simulink model "RBDmodel"  (R2023a)
settings: Solver=ode15s  StartTime=0.0  StopTime=4  FixedStep=0.0001  RelTol=1e-3  AbsTol=1e-3  EnableMultiTasking=on
model workspace (MAT data in the model file):
  C_Gimbal = 0.5
  C_IAP = 0.01
  IAP_Pa = 0
  K_Gimbal = 0
  K_IAP = 200
  LeftAbdominalMuscleForce = 0
  LeftBackMuscleForce = 0
  LeftTransverse1MuscleForce = 0
  LeftTransverse2MuscleForce = 0
  Moment_AR = 0
  Moment_FE = 7.5
  Moment_LB = 0
  RightAbdominalMuscleForce = 0
  RightBackMuscleForce = 0
  RightTransverse1MuscleForce = 0
  RightTransverse2MuscleForce = 0
  a = 1
  b = 1
  muscle_color = [0 0 1]
  muscle_radius = 1
undefined symbols (not defined in the file): X, Y, Z
libraries: nesl_utility x346, sm_lib x329, simulink_extras x33, checkpacklib x3, simulink x1
(part 1 of 12)
settings Model: PacingRate=0.110000  Creator=Siril TD  LastModifiedBy=siril
settings SolverCC: ZeroCrossAlgorithm=Adaptive  AutoInsertRateTranBlk=on
settings DataIOCC: LimitDataPoints=on  MaxDataPoints=50000  ReturnWorkspaceOutputsName=SDOSimTest_Log
settings OptimizationCC: LifeSpan=inf
settings DebuggingCC: IgnoredZcDiagnostic=none  UnconnectedInputMsg=warning  UnconnectedOutputMsg=warning  UnconnectedLineMsg=warning  AllowSymbolicDim=off  SFUnexpectedBacktrackingDiag=warning  SFNoUnconditionalDefaultTransitionDiag=warning  SFExecutionAtInitializationDiag=none  ArithmeticOperatorsInVariantConditions=warning
settings ModelReferenceCC: EnableRefExpFcnMdlSchedulingChecks=on
settings SFSimCC: SimUseLocalCustomCode=off  CustomCodeUndefinedFunction=UseInterfaceOnly
settings RTWCC: RTWUseLocalCustomCode=off  DLArmComputeVersion=19.05
settings CodeAppCC: StateflowObjectComments=on
settings GRTTargetCC: TargetLangStandard=C89/C90 (ANSI)
settings ConfigComp: CovMetricSettings=dw  CovSaveCumulativeToWorkspaceVar=on  CovSaveSingleToWorkspaceVar=on  CovExternalEMLEnable=off  CovSFcnEnable=off
settings SimscapeCC: SimscapeLogType=all  SimscapeLogSimulationStatistics=on  SimscapeLogDataHistory=10000

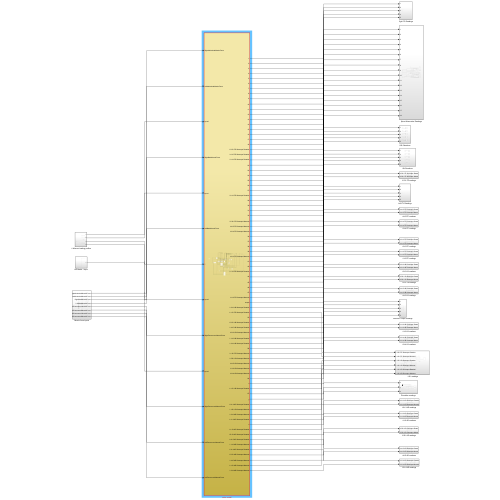
[thumbnail: Simulink's stored preview of the top-level diagram]
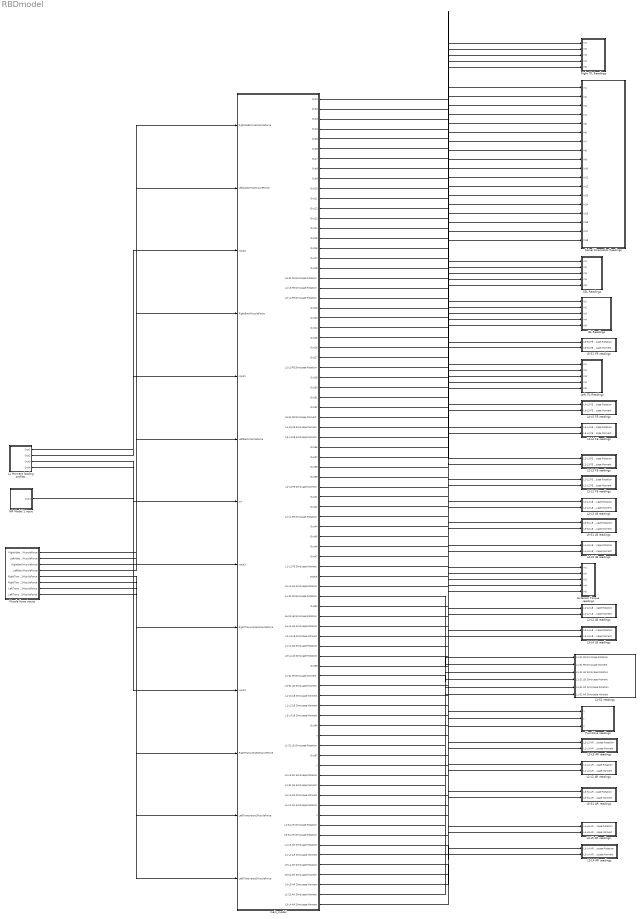
== system RBDmodel ==
  Extensor Torque readings : Subsystem
  IAP Model 1 input : Subsystem
  ISL Readings : Subsystem
  L1 Moment loading profiles : Subsystem
  L1-L2 AR readings : Subsystem
  L1-L2 FE readings : Subsystem
  L1-L2 LB readings : Subsystem
  L1-S1 readings : Subsystem
  L2-L3 AR readings : Subsystem
  L2-L3 FE readings : Subsystem
  L2-L3 LB readings : Subsystem
  L3-L4 AR readings : Subsystem
  L3-L4 FE readings : Subsystem
  L3-L4 LB readings : Subsystem
  L4-L5 AR readings : Subsystem
  L4-L5 FE readings : Subsystem
  L4-L5 LB readings : Subsystem
  L5-S1 AR readings : Subsystem
  L5-S1 FE readings : Subsystem
  L5-S1 LB readings : Subsystem
  Left ITL Readings : Subsystem
  Muscle force inputs : Subsystem
  Plumbline readings : Subsystem
  Right ITL Readings : Subsystem
  SSL Readings : Subsystem
  Spinal Kinematics Readings : Subsystem
  main_model : Subsystem  TreatAsAtomicUnit=on
  wires:
  main_model/20(L4-L5 FE Simscape Rotation) -> L4-L5 FE readings/1(L4-L5 FE Simscape Rotation)
  main_model/67(Out67) -> Extensor Torque readings/5(In5)
  Muscle force inputs/4(LeftBackMuscleForce) -> main_model/6(LeftBackMuscleForce)
  Muscle force inputs/3(RightBackMuscleForce) -> main_model/4(RightBackMuscleForce)
  L1 Moment loading profiles/1(Out1) -> main_model/3(input0)
  main_model/31(Out31) -> SSL Readings/4(In4)
  main_model/81(L1-S1 AR Simscape Moment) -> L1-S1 readings/6(L1-S1 AR Simscape Moment)
  main_model/56(L1-L2 LB Simscape Rotation) -> L1-L2 LB readings/1(L1-L2 LB Simscape Rotation)
  L1 Moment loading profiles/2(Out2) -> main_model/5(input1)
  L1 Moment loading profiles/3(Out3) -> main_model/8(input2)
  main_model/50(L2-L3 LB Simscape Rotation) -> L2-L3 LB readings/1(L2-L3 LB Simscape Rotation)
  main_model/6(Out6) -> SSL Readings/1(In1)
  L1 Moment loading profiles/4(Out4) -> main_model/10(input3)
  Muscle force inputs/1(RightAbdominalMuscleForce) -> main_model/1(RightAbdominalMuscleForce)
  main_model/16(Out16) -> Left ITL Readings/2(In2)
  IAP Model 1 input/1(Out1) -> main_model/7(In7)
  Muscle force inputs/2(LeftAbdominalMuscleForce) -> main_model/2(LeftAbdominalMuscleForce)
  Muscle force inputs/5(RightTransverse1MuscleForce) -> main_model/9(RightTransverse1MuscleForce)
  Muscle force inputs/6(RightTransverse2MuscleForce) -> main_model/11(RightTransverse2MuscleForce)
  main_model/62(L1-L2 LB Simscape Moment) -> L1-L2 LB readings/2(L1-L2 LB Simscape Moment)
  Muscle force inputs/8(LeftTransverse2MuscleForce) -> main_model/13(LeftTransverse2MuscleForce)
  Muscle force inputs/7(LeftTransverse1MuscleForce) -> main_model/12(LeftTransverse1MuscleForce)
  main_model/63(L3-L4 LB Simscape Moment) -> L3-L4 LB readings/2(L3-L4 LB Simscape Moment)
  main_model/1(Out1) -> Spinal Kinematics Readings/1(In1)
  main_model/30(Out30) -> Spinal Kinematics Readings/13(In13)
  main_model/2(Out2) -> Spinal Kinematics Readings/2(In2)
  main_model/13(Out13) -> SSL Readings/2(In2)
  main_model/21(L3-L4 FE Simscape Rotation) -> L3-L4 FE readings/1(L3-L4 FE Simscape Rotation)
  main_model/3(Out3) -> ISL Readings/1(In1)
  main_model/44(Out44) -> Spinal Kinematics Readings/17(In17)
  main_model/25(Out25) -> Spinal Kinematics Readings/11(In11)
  main_model/79(L5-S1 AR Simscape Moment) -> L5-S1 AR readings/2(L5-S1 AR Simscape Moment)
  main_model/4(Out4) -> Spinal Kinematics Readings/3(In3)
  main_model/5(Out5) -> Spinal Kinematics Readings/4(In4)
  main_model/77(L1-L2 AR Simscape Moment) -> L1-L2 AR readings/2(L1-L2 AR Simscape Moment)
  main_model/36(Out36) -> Spinal Kinematics Readings/14(In14)
  main_model/78(L3-L4 AR Simscape Rotation) -> L3-L4 AR readings/1(L3-L4 AR Simscape Rotation)
  main_model/26(Out26) -> Left ITL Readings/3(In3)
  main_model/7(Out7) -> Spinal Kinematics Readings/5(In5)
  main_model/18(Out18) -> Right ITL Readings/3(In3)
  main_model/8(Out8) -> Left ITL Readings/1(In1)
  main_model/9(Out9) -> Right ITL Readings/1(In1)
  main_model/10(Out10) -> Spinal Kinematics Readings/6(In6)
  main_model/11(Out11) -> ISL Readings/2(In2)
  main_model/12(Out12) -> Spinal Kinematics Readings/7(In7)
  main_model/38(Out38) -> Left ITL Readings/4(In4)
  main_model/14(Out14) -> Right ITL Readings/2(In2)
  main_model/15(Out15) -> Spinal Kinematics Readings/8(In8)
  main_model/17(Out17) -> Spinal Kinematics Readings/9(In9)
  main_model/27(Out27) -> Right ITL Readings/4(In4)
  main_model/19(L5-S1 FE Simscape Rotation) -> L5-S1 FE readings/1(L5-S1 FE Simscape Rotation)
  main_model/22(Out22) -> Spinal Kinematics Readings/10(In10)
  main_model/33(L5-S1 FE Simscape Moment) -> L5-S1 FE readings/2(L5-S1 FE Simscape Moment)
  main_model/23(Out23) -> ISL Readings/3(In3)
  main_model/45(Out45) -> Left ITL Readings/5(In5)
  main_model/24(Out24) -> SSL Readings/3(In3)
  main_model/28(L2-L3 FE Simscape Rotation) -> L2-L3 FE readings/1(L2-L3 FE Simscape Rotation)
  main_model/29(Out29) -> Spinal Kinematics Readings/12(In12)
  main_model/32(Out32) -> Right ITL Readings/5(In5)
  main_model/34(L4-L5 FE Simscape Moment) -> L4-L5 FE readings/2(L4-L5 FE Simscape Moment)
  main_model/59(L1-S1 FE Simscape Moment) -> L1-S1 readings/2(L1-S1 FE Simscape Moment)
  main_model/35(L3-L4 FE Simscape Moment) -> L3-L4 FE readings/2(L3-L4 FE Simscape Moment)
  main_model/37(Out37) -> ISL Readings/4(In4)
  main_model/51(L1-S1 FE Simscape Rotation) -> L1-S1 readings/1(L1-S1 FE Simscape Rotation)
  main_model/39(Out39) -> Spinal Kinematics Readings/15(In15)
  main_model/40(L2-L3 FE Simscape Moment) -> L2-L3 FE readings/2(L2-L3 FE Simscape Moment)
  main_model/41(Out41) -> Spinal Kinematics Readings/16(In16)
  main_model/42(Out42) -> SSL Readings/5(In5)
  main_model/43(L1-L2 FE Simscape Rotation) -> L1-L2 FE readings/1(L1-L2 FE Simscape Rotation)
  main_model/46(Out46) -> Spinal Kinematics Readings/18(In18)
  main_model/47(Out47) -> ISL Readings/5(In5)
  main_model/48(L1-L2 FE Simscape Moment) -> L1-L2 FE readings/2(L1-L2 FE Simscape Moment)
  main_model/49(output) -> Extensor Torque readings/1(In1)
  main_model/52(Out52) -> Extensor Torque readings/2(In2)
  main_model/68(y) -> Plumbline readings/2(y)
  main_model/53(L5-S1 LB Simscape Rotation) -> L5-S1 LB readings/1(L5-S1 LB Simscape Rotation)
  main_model/54(L4-L5 LB Simscape Rotation) -> L4-L5 LB readings/1(L4-L5 LB Simscape Rotation)
  main_model/55(L2-L3 LB Simscape Moment) -> L2-L3 LB readings/2(L2-L3 LB Simscape Moment)
  main_model/57(L3-L4 LB Simscape Rotation) -> L3-L4 LB readings/1(L3-L4 LB Simscape Rotation)
  main_model/58(Out58) -> Extensor Torque readings/3(In3)
  main_model/60(L5-S1 LB Simscape Moment) -> L5-S1 LB readings/2(L5-S1 LB Simscape Moment)
  main_model/61(L4-L5 LB Simscape Moment) -> L4-L5 LB readings/2(L4-L5 LB Simscape Moment)
  main_model/64(Out64) -> Extensor Torque readings/4(In4)
  main_model/65(x) -> Plumbline readings/1(x)
  main_model/66(L1-S1 LB Simscape Rotation) -> L1-S1 readings/3(L1-S1 LB Simscape Rotation)
  main_model/69(L2-L3 AR Simscape Rotation) -> L2-L3 AR readings/1(L2-L3 AR Simscape Rotation)
  main_model/70(L1-S1 LB Simscape Moment) -> L1-S1 readings/4(L1-S1 LB Simscape Moment)
  main_model/71(L2-L3 AR Simscape Moment) -> L2-L3 AR readings/2(L2-L3 AR Simscape Moment)
  main_model/72(L1-L2 AR Simscape Rotation) -> L1-L2 AR readings/1(L1-L2 AR Simscape Rotation)
  main_model/73(z) -> Plumbline readings/3(z)
  main_model/74(L1-S1 AR Simscape Rotation) -> L1-S1 readings/5(L1-S1 AR Simscape Rotation)
  main_model/75(L5-S1 AR Simscape Rotation) -> L5-S1 AR readings/1(L5-S1 AR Simscape Rotation)
  main_model/76(L4-L5 AR Simscape Rotation) -> L4-L5 AR readings/1(L4-L5 AR Simscape Rotation)
  main_model/80(L4-L5 AR Simscape Moment) -> L4-L5 AR readings/2(L4-L5 AR Simscape Moment)
  main_model/82(L3-L4 AR Simscape Moment) -> L3-L4 AR readings/2(L3-L4 AR Simscape Moment)

== system RBDmodel/Extensor Torque readings ==
  In1 : Inport
  In2 : Inport  Port=2
  In3 : Inport  Port=3
  In4 : Inport  Port=4
  In5 : Inport  Port=5
  Display{,1..4} (5 alike) : Display
      settings: Decimation=2
  Gain{9,11..14} (5 alike) : Gain
  IAP Extensor Torque at L1-L2 : Scope
  IAP Extensor Torque at L2-L3 (reported) : Scope
  IAP Extensor Torque at L3-L4 : Scope
  IAP Extensor Torque at L4-L5 : Scope
  IAP Extensor Torque at L5-S1 : Scope
  wires:
  Gain11/1 -> Display1/1
  Gain9/1 -> Display/1
  In5/1 -> Gain14/1, IAP Extensor Torque at L5-S1/1
  In2/1 -> Gain9/1, IAP Extensor Torque at L2-L3 (reported)/1
  Gain12/1 -> Display2/1
  In4/1 -> Gain13/1, IAP Extensor Torque at L4-L5/1
  In3/1 -> Gain12/1, IAP Extensor Torque at L3-L4/1
  Gain13/1 -> Display3/1
  In1/1 -> Gain11/1, IAP Extensor Torque at L1-L2/1
  Gain14/1 -> Display4/1

== system RBDmodel/IAP Model 1 input ==
  Constant96 : Constant  Value=IAP_Pa
  Out1 : Outport
  wires:
  Constant96/1 -> Out1/1

== system RBDmodel/ISL Readings ==
  In1 : Inport
  In2 : Inport  Port=2
  In3 : Inport  Port=3
  In4 : Inport  Port=4
  In5 : Inport  Port=5
  L1-L2 ISL force : Scope
  L2-L3 ISL force : Scope
  L3-L4 ISL force : Scope
  L4-L5 ISL force : Scope
  L5-S1 ISL force : Scope
  wires:
  In4/1 -> L5-S1 ISL force/1
  In2/1 -> L2-L3 ISL force/1
  In1/1 -> L1-L2 ISL force/1
  In3/1 -> L3-L4 ISL force/1
  In5/1 -> L4-L5 ISL force/1

== system RBDmodel/L1 Moment loading profiles ==
  Gain10 : Gain  Gain=-1
  Horizontal force at T1 : simulink/Sources/Ramp  slope=0  start=0  InitialOutput=0
  Moment_AR : Sin  Amplitude=Moment_AR  SampleTime=0
  Moment_FE : Sin  Amplitude=-Moment_FE  SampleTime=0
  Moment_LB : Sin  Amplitude=-Moment_LB  SampleTime=0
  Scope2 : Scope
  Out1 : Outport
  Out2 : Outport  Port=2
  Out3 : Outport  Port=3
  Out4 : Outport  Port=4
  wires:
  Gain10/1 -> Scope2/1
  Horizontal force at T1/1 -> Out4/1
  Moment_LB/1 -> Out2/1
  Moment_AR/1 -> Out1/1
  Moment_FE/1 -> Gain10/1, Out3/1

== system RBDmodel/L1-L2 AR readings ==
  L1-L2 AR Simscape Rotation : Inport
  L1-L2 AR Simscape Moment : Inport  Port=2
  L1-L2 AR Moment : Scope
  L1-L2 AR Rotation : Scope
  L1-L2 AR Simscape : Record  FileSettingsInternal="{\"entries\":[{\"content\":{\"excelSettings\":{\"content\":{},\"type\":\"Streamout.ExcelSettings\"}},\"type\":\"Streamout.FileSettingStorage\",\"uuid\":\"b28dc066-991e-4613-a00d-d29ff6d798a1\"}],\"packageUris\":[\"http://schema.mathworks.com/mf0/streamout_blocks/R2020a\"],\"version\":\"1.0\"}"  Layout=[1 1]  SignalsInternal="{\"entries\":[{\"content\":{\"signals\":[{\"content\":{\"blockPath\":[\"RBDmodel/L1-L2 AR readings/L1-L2 AR Simscape\"],\"dimensions\":[1],\"domain\":\"RBDmodel/L1-L2 AR readings/L1-L2 AR Simscape\",\"lineColor\":\"#ff6929\",\"port\":1,\"sid\":[\"\"],\"signalID\":1360,\"signalName\":\"L1-L2 AR Simscape Rotation\"},\"type\":\"RecordBlkView.Signal\",\"uuid\":\"ef38e7f4-5bb5-4ee4-abd3-08050efdce29\"},{\"content\":{\"blockPath\":[\"RBDmodel/L1-L2 AR readings/L1-L2 AR Simscape\"],\"dimensions\":[1],\"domain\":\"RBDmodel/L1-L2 AR readings/L1-L2 AR Simscape\",\"lineColor\":\"#b746ff\",\"port\":2,\"sid\":[\"\"],\"signalID\":1364,\"signalName\":\"L1-L2 AR Simscape Moment\"},\"type\":\"RecordBlkView.Signal\",\"uuid\":\"a5e45ef9-876c-4f21-bd86-513f30723b41\"}]},\"type\":\"RecordBlkView.InputSignals\",\"uuid\":\"1c542607-3eb8-449b-8497-6476f9b5df54\"}],\"packageUris\":[\"http://schema.mathworks.com/mf0/streamout_blocks/R2020a\"],\"version\":\"1.0\"}"  VisualizationBindings="{\"xyplotplugin\":{\"info\":[{\"series\":[],\"subplotID\":1}]}}"  CompatibilityTag=XY
  wires:
  L1-L2 AR Simscape Rotation/1 -> L1-L2 AR Simscape/1, L1-L2 AR Rotation/1
  L1-L2 AR Simscape Moment/1 -> L1-L2 AR Simscape/2, L1-L2 AR Moment/1

== system RBDmodel/L1-L2 FE readings ==
  L1-L2 FE Simscape Rotation : Inport
  L1-L2 FE Simscape Moment : Inport  Port=2
  L1-L2 FE Moment : Scope
  L1-L2 FE Rotation : Scope
  L1-L2 FE Simscape : Record  FileSettingsInternal="{\"entries\":[{\"content\":{\"excelSettings\":{\"content\":{},\"type\":\"Streamout.ExcelSettings\"}},\"type\":\"Streamout.FileSettingStorage\",\"uuid\":\"8ce7ea1e-727d-4085-a2f9-c3a4a6f5bb0a\"}],\"packageUris\":[\"http://schema.mathworks.com/mf0/streamout_blocks/R2020a\"],\"version\":\"1.0\"}"  Layout=[1 1]  SignalsInternal="{\"entries\":[{\"content\":{\"signals\":[{\"content\":{\"blockPath\":[\"RBDmodel/L1-L2 FE readings/L1-L2 FE Simscape\"],\"dimensions\":[1],\"domain\":\"RBDmodel/L1-L2 FE readings/L1-L2 FE Simscape\",\"lineColor\":\"#64d413\",\"port\":1,\"sid\":[\"\"],\"signalID\":1368,\"signalName\":\"L1-L2 FE Simscape Rotation\"},\"type\":\"RecordBlkView.Signal\",\"uuid\":\"45dd78b4-e84e-4b03-8d26-d3924673fb9f\"},{\"content\":{\"blockPath\":[\"RBDmodel/L1-L2 FE readings/L1-L2 FE Simscape\"],\"dimensions\":[1],\"domain\":\"RBDmodel/L1-L2 FE readings/L1-L2 FE Simscape\",\"lineColor\":\"#ff13a6\",\"port\":2,\"sid\":[\"\"],\"signalID\":1372,\"signalName\":\"L1-L2 FE Simscape Moment\"},\"type\":\"RecordBlkView.Signal\",\"uuid\":\"1e4034e5-5361-4be0-a13e-86df1fe44d0f\"}]},\"type\":\"RecordBlkView.InputSignals\",\"uuid\":\"536e5213-b6d8-4f71-bd77-60f8c5ebbdbb\"}],\"packageUris\":[\"http://schema.mathworks.com/mf0/streamout_blocks/R2020a\"],\"version\":\"1.0\"}"  VisualizationBindings="{\"xyplotplugin\":{\"info\":[{\"series\":[],\"subplotID\":1}]}}"  CompatibilityTag=XY
  wires:
  L1-L2 FE Simscape Rotation/1 -> L1-L2 FE Simscape/1, L1-L2 FE Rotation/1
  L1-L2 FE Simscape Moment/1 -> L1-L2 FE Simscape/2, L1-L2 FE Moment/1

== system RBDmodel/L1-L2 LB readings ==
  L1-L2 LB Simscape Rotation : Inport
  L1-L2 LB Simscape Moment : Inport  Port=2
  L1-L2 LB Moment : Scope
  L1-L2 LB Rotation : Scope
  L1-L2 LB Simscape : Record  FileSettingsInternal="{\"entries\":[{\"content\":{\"excelSettings\":{\"content\":{},\"type\":\"Streamout.ExcelSettings\"}},\"type\":\"Streamout.FileSettingStorage\",\"uuid\":\"f91b6da8-1a5e-44a2-9c0b-2edd10b764e6\"}],\"packageUris\":[\"http://schema.mathworks.com/mf0/streamout_blocks/R2020a\"],\"version\":\"1.0\"}"  Layout=[1 1]  SignalsInternal="{\"entries\":[{\"content\":{\"signals\":[{\"content\":{\"blockPath\":[\"RBDmodel/L1-L2 LB readings/L1-L2 LB Simscape\"],\"dimensions\":[1],\"domain\":\"RBDmodel/L1-L2 LB readings/L1-L2 LB Simscape\",\"lineColor\":\"#fe330a\",\"port\":1,\"sid\":[\"\"],\"signalID\":1376,\"signalName\":\"L1-L2 LB Simscape Rotation\"},\"type\":\"RecordBlkView.Signal\",\"uuid\":\"b39e1f2f-f959-4496-b329-aa729bed6301\"},{\"content\":{\"blockPath\":[\"RBDmodel/L1-L2 LB readings/L1-L2 LB Simscape\"],\"dimensions\":[1],\"domain\":\"RBDmodel/L1-L2 LB readings/L1-L2 LB Simscape\",\"lineColor\":\"#22b573\",\"port\":2,\"sid\":[\"\"],\"signalID\":1380,\"signalName\":\"L1-L2 LB Simscape Moment\"},\"type\":\"RecordBlkView.Signal\",\"uuid\":\"c7b78cd7-1479-427e-ae62-48589b678214\"}]},\"type\":\"RecordBlkView.InputSignals\",\"uuid\":\"566f98af-9a37-420a-a360-2b47a0b9b0d7\"}],\"packageUris\":[\"http://schema.mathworks.com/mf0/streamout_blocks/R2020a\"],\"version\":\"1.0\"}"  VisualizationBindings="{\"xyplotplugin\":{\"info\":[{\"series\":[],\"subplotID\":1}]}}"  CompatibilityTag=XY
  wires:
  L1-L2 LB Simscape Moment/1 -> L1-L2 LB Simscape/2, L1-L2 LB Moment/1
  L1-L2 LB Simscape Rotation/1 -> L1-L2 LB Simscape/1, L1-L2 LB Rotation/1

== system RBDmodel/L1-S1 readings ==
  L1-S1 FE Simscape Rotation : Inport
  L1-S1 FE Simscape Moment : Inport  Port=2
  L1-S1 LB Simscape Rotation : Inport  Port=3
  L1-S1 LB Simscape Moment : Inport  Port=4
  L1-S1 AR Simscape Rotation : Inport  Port=5
  L1-S1 AR Simscape Moment : Inport  Port=6
  Check Flexion Angle : checkpacklib/Check Custom Bounds  InstantiateOnLoad=on  enabled=off  stopWhenAssertionFail=off  export=off  ViewDlgPos=[100 200 510 390]  OpenViewOnLoad=off  LaunchViewOnOpen=off  TimeUnits=seconds  EnableUpperBound=on  UpperBoundTimes=[5 10]  UpperBoundAmplitudes=[51 51];  EnableLowerBound=on  LowerBoundTimes=[6 10]  LowerBoundAmplitudes=[49 49];
      settings: LibrarySourceBlock=sdolib/Signal Constraints/Check Custom Bounds
  L1-S1 AR Rotation : Scope
  L1-S1 AR Simscape : Record  FileSettingsInternal="{\"entries\":[{\"content\":{\"excelSettings\":{\"content\":{},\"type\":\"Streamout.ExcelSettings\"}},\"type\":\"Streamout.FileSettingStorage\",\"uuid\":\"b954e3b6-b992-4288-8e9e-83c0e0eed84f\"}],\"packageUris\":[\"http://schema.mathworks.com/mf0/streamout_blocks/R2020a\"],\"version\":\"1.0\"}"  Layout=[1 1]  SignalsInternal="{\"entries\":[{\"content\":{\"signals\":[{\"content\":{\"blockPath\":[\"RBDmodel/L1-S1 readings/L1-S1 AR Simscape\"],\"dimensions\":[1,1],\"domain\":\"RBDmodel/L1-S1 readings/L1-S1 AR Simscape\",\"lineColor\":\"#edb120\",\"port\":1,\"sid\":[\"\"],\"signalID\":1392,\"signalName\":\"L1-S1 AR Simscape Rotation\"},\"type\":\"RecordBlkView.Signal\",\"uuid\":\"abf6d3a3-333d-4b08-b552-24fefc0574f8\"},{\"content\":{\"blockPath\":[\"RBDmodel/L1-S1 readings/L1-S1 AR Simscape\"],\"dimensions\":[1],\"domain\":\"RBDmodel/L1-S1 readings/L1-S1 AR Simscape\",\"lineColor\":\"#7e2f8e\",\"port\":2,\"sid\":[\"\"],\"signalID\":1396,\"signalName\":\"L1-S1 AR Simscape Moment\"},\"type\":\"RecordBlkView.Signal\",\"uuid\":\"43efc21e-c542-4766-995d-39dc3de40fa3\"}]},\"type\":\"RecordBlkView.InputSignals\",\"uuid\":\"e7fd8fa1-e77d-4e34-884c-9c18986ac726\"}],\"packageUris\":[\"http://schema.mathworks.com/mf0/streamout_blocks/R2020a\"],\"version\":\"1.0\"}"  VisualizationBindings="{\"xyplotplugin\":{\"info\":[{\"series\":[],\"subplotID\":1}]}}"  CompatibilityTag=XY
  L1-S1 AR when LB loading : Record  FileSettingsInternal="{\"entries\":[{\"content\":{\"excelSettings\":{\"content\":{},\"type\":\"Streamout.ExcelSettings\"}},\"type\":\"Streamout.FileSettingStorage\",\"uuid\":\"7c9a55b9-26e2-4dee-8ab6-75e3d662341a\"}],\"packageUris\":[\"http://schema.mathworks.com/mf0/streamout_blocks/R2020a\"],\"version\":\"1.0\"}"  Layout=[1 1]  SignalsInternal="{\"entries\":[{\"content\":{\"signals\":[{\"content\":{\"blockPath\":[\"RBDmodel/L1-S1 readings/L1-S1 AR when LB loading\"],\"dimensions\":[1,1],\"domain\":\"RBDmodel/L1-S1 readings/L1-S1 AR when LB loading\",\"lineColor\":\"#77ac30\",\"port\":1,\"sid\":[\"\"],\"signalID\":1400,\"signalName\":\"L1-S1 AR Simscape Rotation\"},\"type\":\"RecordBlkView.Signal\",\"uuid\":\"01449e03-afe1-494b-a7bb-817c1e7535e4\"},{\"content\":{\"blockPath\":[\"RBDmodel/L1-S1 readings/L1-S1 AR when LB loading\"],\"dimensions\":[1],\"domain\":\"RBDmodel/L1-S1 readings/L1-S1 AR when LB loading\",\"lineColor\":\"#4dbeee\",\"port\":2,\"sid\":[\"\"],\"signalID\":1404,\"signalName\":\"L1-S1 LB Simscape Moment\"},\"type\":\"RecordBlkView.Signal\",\"uuid\":\"edd20f08-c703-4c4e-842e-61ae2f12c9d8\"}]},\"type\":\"RecordBlkView.InputSignals\",\"uuid\":\"629facc2-2845-4351-bc8b-8e4e78e1c50b\"}],\"packageUris\":[\"http://schema.mathworks.com/mf0/streamout_blocks/R2020a\"],\"version\":\"1.0\"}"  VisualizationBindings="{\"xyplotplugin\":{\"info\":[{\"series\":[],\"subplotID\":1}]}}"  CompatibilityTag=XY
  L1-S1 FE Rotation : Scope
  L1-S1 FE Simscape : Record  FileSettingsInternal="{\"entries\":[{\"content\":{\"excelSettings\":{\"content\":{},\"type\":\"Streamout.ExcelSettings\"}},\"type\":\"Streamout.FileSettingStorage\",\"uuid\":\"4277ec63-d6bc-434d-a603-e60f5b770cfc\"}],\"packageUris\":[\"http://schema.mathworks.com/mf0/streamout_blocks/R2020a\"],\"version\":\"1.0\"}"  Layout=[1 1]  SignalsInternal="{\"entries\":[{\"content\":{\"signals\":[{\"content\":{\"blockPath\":[\"RBDmodel/L1-S1 readings/L1-S1 FE Simscape\"],\"dimensions\":[1,1],\"domain\":\"RBDmodel/L1-S1 readings/L1-S1 FE Simscape\",\"lineColor\":\"#0072bd\",\"port\":1,\"sid\":[\"\"],\"signalID\":1384,\"signalName\":\"L1-S1 FE Simscape Rotation\"},\"type\":\"RecordBlkView.Signal\",\"uuid\":\"ecd61b72-090b-489d-8864-b303b80e918f\"},{\"content\":{\"blockPath\":[\"RBDmodel/L1-S1 readings/L1-S1 FE Simscape\"],\"dimensions\":[1],\"domain\":\"RBDmodel/L1-S1 readings/L1-S1 FE Simscape\",\"lineColor\":\"#d95319\",\"port\":2,\"sid\":[\"\"],\"signalID\":1388,\"signalName\":\"L1-S1 FE Simscape Moment\"},\"type\":\"RecordBlkView.Signal\",\"uuid\":\"76b91155-e619-4f04-befa-9af8b9c1bafd\"}]},\"type\":\"RecordBlkView.InputSignals\",\"uuid\":\"ae4eb2e1-11d8-4584-857d-70c1fe6f9d4a\"}],\"packageUris\":[\"http://schema.mathworks.com/mf0/streamout_blocks/R2020a\"],\"version\":\"1.0\"}"  VisualizationBindings="{\"xyplotplugin\":{\"info\":[{\"series\":[],\"subplotID\":1}]}}"  CompatibilityTag=XY
  L1-S1 LB Rotation : Scope
  L1-S1 LB Simscape : Record  FileSettingsInternal="{\"entries\":[{\"content\":{\"excelSettings\":{\"content\":{},\"type\":\"Streamout.ExcelSettings\"}},\"type\":\"Streamout.FileSettingStorage\",\"uuid\":\"d051a5cc-fb2e-466c-bd05-561f4ba50a96\"}],\"packageUris\":[\"http://schema.mathworks.com/mf0/streamout_blocks/R2020a\"],\"version\":\"1.0\"}"  Layout=[1 1]  SignalsInternal="{\"entries\":[{\"content\":{\"signals\":[{\"content\":{\"blockPath\":[\"RBDmodel/L1-S1 readings/L1-S1 LB Simscape\"],\"dimensions\":[1,1],\"domain\":\"RBDmodel/L1-S1 readings/L1-S1 LB Simscape\",\"lineColor\":\"#a2142f\",\"port\":1,\"sid\":[\"\"],\"signalID\":1408,\"signalName\":\"L1-S1 LB Simscape Rotation\"},\"type\":\"RecordBlkView.Signal\",\"uuid\":\"7dd0c97e-21b8-44c0-8611-8b75f369b7ab\"},{\"content\":{\"blockPath\":[\"RBDmodel/L1-S1 readings/L1-S1 LB Simscape\"],\"dimensions\":[1],\"domain\":\"RBDmodel/L1-S1 readings/L1-S1 LB Simscape\",\"lineColor\":\"#139fff\",\"port\":2,\"sid\":[\"\"],\"signalID\":1412,\"signalName\":\"L1-S1 LB Simscape Moment\"},\"type\":\"RecordBlkView.Signal\",\"uuid\":\"cd7abbff-07eb-403b-8bd0-ef6e2fd2e77a\"}]},\"type\":\"RecordBlkView.InputSignals\",\"uuid\":\"e04c7294-0c2c-4555-ba51-1b5841c30b05\"}],\"packageUris\":[\"http://schema.mathworks.com/mf0/streamout_blocks/R2020a\"],\"version\":\"1.0\"}"  VisualizationBindings="{\"xyplotplugin\":{\"info\":[{\"series\":[],\"subplotID\":1}]}}"  CompatibilityTag=XY
  wires:
  L1-S1 LB Simscape Rotation/1 -> L1-S1 LB Simscape/1, L1-S1 LB Rotation/1
  L1-S1 FE Simscape Rotation/1 -> Check Flexion Angle/1, L1-S1 FE Rotation/1, L1-S1 FE Simscape/1
  L1-S1 AR Simscape Rotation/1 -> L1-S1 AR when LB loading/1, L1-S1 AR Rotation/1, L1-S1 AR Simscape/1
  L1-S1 LB Simscape Moment/1 -> L1-S1 LB Simscape/2, L1-S1 AR when LB loading/2
  L1-S1 FE Simscape Moment/1 -> L1-S1 FE Simscape/2
  L1-S1 AR Simscape Moment/1 -> L1-S1 AR Simscape/2

== system RBDmodel/L2-L3 AR readings ==
  L2-L3 AR Simscape Rotation : Inport
  L2-L3 AR Simscape Moment : Inport  Port=2
  L2-L3 AR Moment : Scope
  L2-L3 AR Rotation : Scope
  L2-L3 AR Simscape : Record  FileSettingsInternal="{\"entries\":[{\"content\":{\"excelSettings\":{\"content\":{},\"type\":\"Streamout.ExcelSettings\"}},\"type\":\"Streamout.FileSettingStorage\",\"uuid\":\"1b3dca45-e25d-4c43-83f1-4bff6aa87f96\"}],\"packageUris\":[\"http://schema.mathworks.com/mf0/streamout_blocks/R2020a\"],\"version\":\"1.0\"}"  Layout=[1 1]  SignalsInternal="{\"entries\":[{\"content\":{\"signals\":[{\"content\":{\"blockPath\":[\"RBDmodel/L2-L3 AR readings/L2-L3 AR Simscape\"],\"dimensions\":[1],\"domain\":\"RBDmodel/L2-L3 AR readings/L2-L3 AR Simscape\",\"lineColor\":\"#ff6929\",\"port\":1,\"sid\":[\"\"],\"signalID\":1416,\"signalName\":\"L2-L3 AR Simscape Rotation\"},\"type\":\"RecordBlkView.Signal\",\"uuid\":\"6cc8f0af-e808-4452-a883-93ff95b6691d\"},{\"content\":{\"blockPath\":[\"RBDmodel/L2-L3 AR readings/L2-L3 AR Simscape\"],\"dimensions\":[1],\"domain\":\"RBDmodel/L2-L3 AR readings/L2-L3 AR Simscape\",\"lineColor\":\"#b746ff\",\"port\":2,\"sid\":[\"\"],\"signalID\":1420,\"signalName\":\"L2-L3 AR Simscape Moment\"},\"type\":\"RecordBlkView.Signal\",\"uuid\":\"ff3d70a9-4564-486c-aba3-cac8b714e595\"}]},\"type\":\"RecordBlkView.InputSignals\",\"uuid\":\"eee5028e-58a0-4755-b03d-c014803a4ea2\"}],\"packageUris\":[\"http://schema.mathworks.com/mf0/streamout_blocks/R2020a\"],\"version\":\"1.0\"}"  VisualizationBindings="{\"xyplotplugin\":{\"info\":[{\"series\":[],\"subplotID\":1}]}}"  CompatibilityTag=XY
  wires:
  L2-L3 AR Simscape Rotation/1 -> L2-L3 AR Simscape/1, L2-L3 AR Rotation/1
  L2-L3 AR Simscape Moment/1 -> L2-L3 AR Simscape/2, L2-L3 AR Moment/1

== system RBDmodel/L2-L3 FE readings ==
  L2-L3 FE Simscape Rotation : Inport
  L2-L3 FE Simscape Moment : Inport  Port=2
  L2-L3 FE Moment : Scope
  L2-L3 FE Rotation : Scope
  L2-L3 FE Simscape : Record  FileSettingsInternal="{\"entries\":[{\"content\":{\"excelSettings\":{\"content\":{},\"type\":\"Streamout.ExcelSettings\"}},\"type\":\"Streamout.FileSettingStorage\",\"uuid\":\"a8dbeb5b-ff1f-49c5-807a-ed83070a13e0\"}],\"packageUris\":[\"http://schema.mathworks.com/mf0/streamout_blocks/R2020a\"],\"version\":\"1.0\"}"  Layout=[1 1]  SignalsInternal="{\"entries\":[{\"content\":{\"signals\":[{\"content\":{\"blockPath\":[\"RBDmodel/L2-L3 FE readings/L2-L3 FE Simscape\"],\"dimensions\":[1],\"domain\":\"RBDmodel/L2-L3 FE readings/L2-L3 FE Simscape\",\"lineColor\":\"#64d413\",\"port\":1,\"sid\":[\"\"],\"signalID\":1424,\"signalName\":\"L2-L3 FE Simscape Rotation\"},\"type\":\"RecordBlkView.Signal\",\"uuid\":\"267323ca-974f-4cd0-975f-d21e9ee7cdb8\"},{\"content\":{\"blockPath\":[\"RBDmodel/L2-L3 FE readings/L2-L3 FE Simscape\"],\"dimensions\":[1],\"domain\":\"RBDmodel/L2-L3 FE readings/L2-L3 FE Simscape\",\"lineColor\":\"#ff13a6\",\"port\":2,\"sid\":[\"\"],\"signalID\":1428,\"signalName\":\"L2-L3 FE Simscape Moment\"},\"type\":\"RecordBlkView.Signal\",\"uuid\":\"9512b6ba-45f0-4364-9c80-9ca55313e08f\"}]},\"type\":\"RecordBlkView.InputSignals\",\"uuid\":\"4b10e0a9-aa08-416c-827e-f4abb51435b0\"}],\"packageUris\":[\"http://schema.mathworks.com/mf0/streamout_blocks/R2020a\"],\"version\":\"1.0\"}"  VisualizationBindings="{\"xyplotplugin\":{\"info\":[{\"series\":[],\"subplotID\":1}]}}"  CompatibilityTag=XY
  wires:
  L2-L3 FE Simscape Rotation/1 -> L2-L3 FE Simscape/1, L2-L3 FE Rotation/1
  L2-L3 FE Simscape Moment/1 -> L2-L3 FE Simscape/2, L2-L3 FE Moment/1

== system RBDmodel/L2-L3 LB readings ==
  L2-L3 LB Simscape Rotation : Inport
  L2-L3 LB Simscape Moment : Inport  Port=2
  L2-L3 LB Moment : Scope
  L2-L3 LB Rotation : Scope
  L2-L3 LB Simscape : Record  FileSettingsInternal="{\"entries\":[{\"content\":{\"excelSettings\":{\"content\":{},\"type\":\"Streamout.ExcelSettings\"}},\"type\":\"Streamout.FileSettingStorage\",\"uuid\":\"ebb8c812-f4e5-4f1b-bb26-5cc9383d42b0\"}],\"packageUris\":[\"http://schema.mathworks.com/mf0/streamout_blocks/R2020a\"],\"version\":\"1.0\"}"  Layout=[1 1]  SignalsInternal="{\"entries\":[{\"content\":{\"signals\":[{\"content\":{\"blockPath\":[\"RBDmodel/L2-L3 LB readings/L2-L3 LB Simscape\"],\"dimensions\":[1],\"domain\":\"RBDmodel/L2-L3 LB readings/L2-L3 LB Simscape\",\"lineColor\":\"#fe330a\",\"port\":1,\"sid\":[\"\"],\"signalID\":1432,\"signalName\":\"L2-L3 LB Simscape Rotation\"},\"type\":\"RecordBlkView.Signal\",\"uuid\":\"0fb72d85-b961-4ead-bd0f-95fcc3cebcfa\"},{\"content\":{\"blockPath\":[\"RBDmodel/L2-L3 LB readings/L2-L3 LB Simscape\"],\"dimensions\":[1],\"domain\":\"RBDmodel/L2-L3 LB readings/L2-L3 LB Simscape\",\"lineColor\":\"#22b573\",\"port\":2,\"sid\":[\"\"],\"signalID\":1436,\"signalName\":\"L2-L3 LB Simscape Moment\"},\"type\":\"RecordBlkView.Signal\",\"uuid\":\"42bc87f5-2a0c-4979-a0da-e5eb35a423cd\"}]},\"type\":\"RecordBlkView.InputSignals\",\"uuid\":\"041227a4-07e5-4f5e-b607-d8ebf8f118c5\"}],\"packageUris\":[\"http://schema.mathworks.com/mf0/streamout_blocks/R2020a\"],\"version\":\"1.0\"}"  VisualizationBindings="{\"xyplotplugin\":{\"info\":[{\"series\":[],\"subplotID\":1}]}}"  CompatibilityTag=XY
  wires:
  L2-L3 LB Simscape Rotation/1 -> L2-L3 LB Simscape/1, L2-L3 LB Rotation/1
  L2-L3 LB Simscape Moment/1 -> L2-L3 LB Simscape/2, L2-L3 LB Moment/1

== system RBDmodel/L3-L4 AR readings ==
  L3-L4 AR Simscape Rotation : Inport
  L3-L4 AR Simscape Moment : Inport  Port=2
  L3-L4 AR Moment : Scope
  L3-L4 AR Rotation : Scope
  L3-L4 AR Simscape : Record  FileSettingsInternal="{\"entries\":[{\"content\":{\"excelSettings\":{\"content\":{},\"type\":\"Streamout.ExcelSettings\"}},\"type\":\"Streamout.FileSettingStorage\",\"uuid\":\"0d852f55-8e65-459e-b217-a04e03d20f27\"}],\"packageUris\":[\"http://schema.mathworks.com/mf0/streamout_blocks/R2020a\"],\"version\":\"1.0\"}"  Layout=[1 1]  SignalsInternal="{\"entries\":[{\"content\":{\"signals\":[{\"content\":{\"blockPath\":[\"RBDmodel/L3-L4 AR readings/L3-L4 AR Simscape\"],\"dimensions\":[1],\"domain\":\"RBDmodel/L3-L4 AR readings/L3-L4 AR Simscape\",\"lineColor\":\"#0072bd\",\"port\":1,\"sid\":[\"\"],\"signalID\":1440,\"signalName\":\"L3-L4 AR Simscape Rotation\"},\"type\":\"RecordBlkView.Signal\",\"uuid\":\"ab78c45a-22f3-4be6-82c1-21e7edc07753\"},{\"content\":{\"blockPath\":[\"RBDmodel/L3-L4 AR readings/L3-L4 AR Simscape\"],\"dimensions\":[1],\"domain\":\"RBDmodel/L3-L4 AR readings/L3-L4 AR Simscape\",\"lineColor\":\"#d95319\",\"port\":2,\"sid\":[\"\"],\"signalID\":1444,\"signalName\":\"L3-L4 AR Simscape Moment\"},\"type\":\"RecordBlkView.Signal\",\"uuid\":\"17c22d22-07ea-4150-83f9-a9eeae99386d\"}]},\"type\":\"RecordBlkView.InputSignals\",\"uuid\":\"b3558f42-164e-48d0-a33e-bbd3c8029686\"}],\"packageUris\":[\"http://schema.mathworks.com/mf0/streamout_blocks/R2020a\"],\"version\":\"1.0\"}"  VisualizationBindings="{\"xyplotplugin\":{\"info\":[{\"series\":[],\"subplotID\":1}]}}"  CompatibilityTag=XY
  wires:
  L3-L4 AR Simscape Rotation/1 -> L3-L4 AR Simscape/1, L3-L4 AR Rotation/1
  L3-L4 AR Simscape Moment/1 -> L3-L4 AR Simscape/2, L3-L4 AR Moment/1

== system RBDmodel/L3-L4 FE readings ==
  L3-L4 FE Simscape Rotation : Inport
  L3-L4 FE Simscape Moment : Inport  Port=2
  L3-L4 FE Moment : Scope
  L3-L4 FE Rotation : Scope
  L3-L4 FE Simscape : Record  FileSettingsInternal="{\"entries\":[{\"content\":{\"excelSettings\":{\"content\":{},\"type\":\"Streamout.ExcelSettings\"}},\"type\":\"Streamout.FileSettingStorage\",\"uuid\":\"4a97007c-b2c5-4a2b-a22c-db91ba4f89a2\"}],\"packageUris\":[\"http://schema.mathworks.com/mf0/streamout_blocks/R2020a\"],\"version\":\"1.0\"}"  Layout=[1 1]  SignalsInternal="{\"entries\":[{\"content\":{\"signals\":[{\"content\":{\"blockPath\":[\"RBDmodel/L3-L4 FE readings/L3-L4 FE Simscape\"],\"dimensions\":[1],\"domain\":\"RBDmodel/L3-L4 FE readings/L3-L4 FE Simscape\",\"lineColor\":\"#edb120\",\"port\":1,\"sid\":[\"\"],\"signalID\":1448,\"signalName\":\"L3-L4 FE Simscape Rotation\"},\"type\":\"RecordBlkView.Signal\",\"uuid\":\"7d4d5f63-98ed-4c33-a68e-7ea08ee81c3e\"},{\"content\":{\"blockPath\":[\"RBDmodel/L3-L4 FE readings/L3-L4 FE Simscape\"],\"dimensions\":[1],\"domain\":\"RBDmodel/L3-L4 FE readings/L3-L4 FE Simscape\",\"lineColor\":\"#7e2f8e\",\"port\":2,\"sid\":[\"\"],\"signalID\":1452,\"signalName\":\"L3-L4 FE Simscape Moment\"},\"type\":\"RecordBlkView.Signal\",\"uuid\":\"73302c47-25cf-45c0-afae-838eeb6d55fc\"}]},\"type\":\"RecordBlkView.InputSignals\",\"uuid\":\"5f96cd38-8400-44a5-addf-73c7b57d19bc\"}],\"packageUris\":[\"http://schema.mathworks.com/mf0/streamout_blocks/R2020a\"],\"version\":\"1.0\"}"  VisualizationBindings="{\"xyplotplugin\":{\"info\":[{\"series\":[],\"subplotID\":1}]}}"  CompatibilityTag=XY
  wires:
  L3-L4 FE Simscape Rotation/1 -> L3-L4 FE Simscape/1, L3-L4 FE Rotation/1
  L3-L4 FE Simscape Moment/1 -> L3-L4 FE Simscape/2, L3-L4 FE Moment/1

== system RBDmodel/L3-L4 LB readings ==
  L3-L4 LB Simscape Rotation : Inport
  L3-L4 LB Simscape Moment : Inport  Port=2
  L3-L4 LB Moment : Scope
  L3-L4 LB Rotation : Scope
  L3-L4 LB Simscape : Record  FileSettingsInternal="{\"entries\":[{\"content\":{\"excelSettings\":{\"content\":{},\"type\":\"Streamout.ExcelSettings\"}},\"type\":\"Streamout.FileSettingStorage\",\"uuid\":\"1c058524-eb60-4b6f-8fef-1b5d5278ec82\"}],\"packageUris\":[\"http://schema.mathworks.com/mf0/streamout_blocks/R2020a\"],\"version\":\"1.0\"}"  Layout=[1 1]  SignalsInternal="{\"entries\":[{\"content\":{\"signals\":[{\"content\":{\"blockPath\":[\"RBDmodel/L3-L4 LB readings/L3-L4 LB Simscape\"],\"dimensions\":[1],\"domain\":\"RBDmodel/L3-L4 LB readings/L3-L4 LB Simscape\",\"lineColor\":\"#77ac30\",\"port\":1,\"sid\":[\"\"],\"signalID\":1456,\"signalName\":\"L3-L4 LB Simscape Rotation\"},\"type\":\"RecordBlkView.Signal\",\"uuid\":\"5a739d62-33a5-4aef-9607-495665c9ce2b\"},{\"content\":{\"blockPath\":[\"RBDmodel/L3-L4 LB readings/L3-L4 LB Simscape\"],\"dimensions\":[1],\"domain\":\"RBDmodel/L3-L4 LB readings/L3-L4 LB Simscape\",\"lineColor\":\"#4dbeee\",\"port\":2,\"sid\":[\"\"],\"signalID\":1460,\"signalName\":\"L3-L4 LB Simscape Moment\"},\"type\":\"RecordBlkView.Signal\",\"uuid\":\"9e617853-7615-4851-8a2c-99ab70baefe5\"}]},\"type\":\"RecordBlkView.InputSignals\",\"uuid\":\"b25987bc-9b31-4f4e-84c6-06133afb0f97\"}],\"packageUris\":[\"http://schema.mathworks.com/mf0/streamout_blocks/R2020a\"],\"version\":\"1.0\"}"  VisualizationBindings="{\"xyplotplugin\":{\"info\":[{\"series\":[],\"subplotID\":1}]}}"  CompatibilityTag=XY
  wires:
  L3-L4 LB Simscape Rotation/1 -> L3-L4 LB Simscape/1, L3-L4 LB Rotation/1
  L3-L4 LB Simscape Moment/1 -> L3-L4 LB Simscape/2, L3-L4 LB Moment/1

== system RBDmodel/L4-L5 AR readings ==
  L4-L5 AR Simscape Rotation : Inport
  L4-L5 AR Simscape Moment : Inport  Port=2
  L4-L5 AR Moment : Scope
  L4-L5 AR Rotation : Scope
  L4-L5 AR Simscape : Record  FileSettingsInternal="{\"entries\":[{\"content\":{\"excelSettings\":{\"content\":{},\"type\":\"Streamout.ExcelSettings\"}},\"type\":\"Streamout.FileSettingStorage\",\"uuid\":\"22ee5429-b0dc-4563-83b8-15fc97b18f1f\"}],\"packageUris\":[\"http://schema.mathworks.com/mf0/streamout_blocks/R2020a\"],\"version\":\"1.0\"}"  Layout=[1 1]  SignalsInternal="{\"entries\":[{\"content\":{\"signals\":[{\"content\":{\"blockPath\":[\"RBDmodel/L4-L5 AR readings/L4-L5 AR Simscape\"],\"dimensions\":[1],\"domain\":\"RBDmodel/L4-L5 AR readings/L4-L5 AR Simscape\",\"lineColor\":\"#a2142f\",\"port\":1,\"sid\":[\"\"],\"signalID\":1464,\"signalName\":\"L4-L5 AR Simscape Rotation\"},\"type\":\"RecordBlkView.Signal\",\"uuid\":\"0ca04219-1675-4bf3-aaf7-5de8f3f36567\"},{\"content\":{\"blockPath\":[\"RBDmodel/L4-L5 AR readings/L4-L5 AR Simscape\"],\"dimensions\":[1],\"domain\":\"RBDmodel/L4-L5 AR readings/L4-L5 AR Simscape\",\"lineColor\":\"#139fff\",\"port\":2,\"sid\":[\"\"],\"signalID\":1468,\"signalName\":\"L4-L5 AR Simscape Moment\"},\"type\":\"RecordBlkView.Signal\",\"uuid\":\"c382802c-b30d-4af3-bfb8-7039867d3d57\"}]},\"type\":\"RecordBlkView.InputSignals\",\"uuid\":\"f0d5fbce-0274-4ae0-9542-7125bf43316b\"}],\"packageUris\":[\"http://schema.mathworks.com/mf0/streamout_blocks/R2020a\"],\"version\":\"1.0\"}"  VisualizationBindings="{\"xyplotplugin\":{\"info\":[{\"series\":[],\"subplotID\":1}]}}"  CompatibilityTag=XY
  wires:
  L4-L5 AR Simscape Moment/1 -> L4-L5 AR Simscape/2, L4-L5 AR Moment/1
  L4-L5 AR Simscape Rotation/1 -> L4-L5 AR Simscape/1, L4-L5 AR Rotation/1

== system RBDmodel/L4-L5 FE readings ==
  L4-L5 FE Simscape Rotation : Inport
  L4-L5 FE Simscape Moment : Inport  Port=2
  L4-L5 FE Moment : Scope
  L4-L5 FE Rotation : Scope
  L4-L5 FE Simscape : Record  FileSettingsInternal="{\"entries\":[{\"content\":{\"excelSettings\":{\"content\":{},\"type\":\"Streamout.ExcelSettings\"}},\"type\":\"Streamout.FileSettingStorage\",\"uuid\":\"f454a2f2-99ca-4f18-a30c-f3205bc0580a\"}],\"packageUris\":[\"http://schema.mathworks.com/mf0/streamout_blocks/R2020a\"],\"version\":\"1.0\"}"  Layout=[1 1]  SignalsInternal="{\"entries\":[{\"content\":{\"signals\":[{\"content\":{\"blockPath\":[\"RBDmodel/L4-L5 FE readings/L4-L5 FE Simscape\"],\"dimensions\":[1],\"domain\":\"RBDmodel/L4-L5 FE readings/L4-L5 FE Simscape\",\"lineColor\":\"#ff6929\",\"port\":1,\"sid\":[\"\"],\"signalID\":1472,\"signalName\":\"L4-L5 FE Simscape Rotation\"},\"type\":\"RecordBlkView.Signal\",\"uuid\":\"fc1770ed-59ca-4c60-9fc3-df78d3bca789\"},{\"content\":{\"blockPath\":[\"RBDmodel/L4-L5 FE readings/L4-L5 FE Simscape\"],\"dimensions\":[1],\"domain\":\"RBDmodel/L4-L5 FE readings/L4-L5 FE Simscape\",\"lineColor\":\"#b746ff\",\"port\":2,\"sid\":[\"\"],\"signalID\":1476,\"signalName\":\"L4-L5 FE Simscape Moment\"},\"type\":\"RecordBlkView.Signal\",\"uuid\":\"7c720adf-74bd-4475-8954-e54a6efb346b\"}]},\"type\":\"RecordBlkView.InputSignals\",\"uuid\":\"44936656-2524-4106-9aff-c12a018b7abf\"}],\"packageUris\":[\"http://schema.mathworks.com/mf0/streamout_blocks/R2020a\"],\"version\":\"1.0\"}"  VisualizationBindings="{\"xyplotplugin\":{\"info\":[{\"series\":[],\"subplotID\":1}]}}"  CompatibilityTag=XY
  wires:
  L4-L5 FE Simscape Rotation/1 -> L4-L5 FE Simscape/1, L4-L5 FE Rotation/1
  L4-L5 FE Simscape Moment/1 -> L4-L5 FE Simscape/2, L4-L5 FE Moment/1

== system RBDmodel/L4-L5 LB readings ==
  L4-L5 LB Simscape Rotation : Inport
  L4-L5 LB Simscape Moment : Inport  Port=2
  L4-L5 LB Moment : Scope
  L4-L5 LB Rotation : Scope
  L4-L5 LB Simscape : Record  FileSettingsInternal="{\"entries\":[{\"content\":{\"excelSettings\":{\"content\":{},\"type\":\"Streamout.ExcelSettings\"}},\"type\":\"Streamout.FileSettingStorage\",\"uuid\":\"bb960ea0-e781-41a9-8e2d-b5d562a32fcc\"}],\"packageUris\":[\"http://schema.mathworks.com/mf0/streamout_blocks/R2020a\"],\"version\":\"1.0\"}"  Layout=[1 1]  SignalsInternal="{\"entries\":[{\"content\":{\"signals\":[{\"content\":{\"blockPath\":[\"RBDmodel/L4-L5 LB readings/L4-L5 LB Simscape\"],\"dimensions\":[1],\"domain\":\"RBDmodel/L4-L5 LB readings/L4-L5 LB Simscape\",\"lineColor\":\"#64d413\",\"port\":1,\"sid\":[\"\"],\"signalID\":1480,\"signalName\":\"L4-L5 LB Simscape Rotation\"},\"type\":\"RecordBlkView.Signal\",\"uuid\":\"b7d969e9-e827-4d29-92bf-40f9a8d059a7\"},{\"content\":{\"blockPath\":[\"RBDmodel/L4-L5 LB readings/L4-L5 LB Simscape\"],\"dimensions\":[1],\"domain\":\"RBDmodel/L4-L5 LB readings/L4-L5 LB Simscape\",\"lineColor\":\"#ff13a6\",\"port\":2,\"sid\":[\"\"],\"signalID\":1484,\"signalName\":\"L4-L5 LB Simscape Moment\"},\"type\":\"RecordBlkView.Signal\",\"uuid\":\"98a4c43d-595b-402d-9839-dc805f07583d\"}]},\"type\":\"RecordBlkView.InputSignals\",\"uuid\":\"a863a4c4-920c-4be8-b620-d76d13961c7a\"}],\"packageUris\":[\"http://schema.mathworks.com/mf0/streamout_blocks/R2020a\"],\"version\":\"1.0\"}"  VisualizationBindings="{\"xyplotplugin\":{\"info\":[{\"series\":[],\"subplotID\":1}]}}"  CompatibilityTag=XY
  wires:
  L4-L5 LB Simscape Moment/1 -> L4-L5 LB Simscape/2, L4-L5 LB Moment/1
  L4-L5 LB Simscape Rotation/1 -> L4-L5 LB Simscape/1, L4-L5 LB Rotation/1

== system RBDmodel/L5-S1 AR readings ==
  L5-S1 AR Simscape Rotation : Inport
  L5-S1 AR Simscape Moment : Inport  Port=2
  L5-S1 AR Moment : Scope
  L5-S1 AR Rotation : Scope
  L5-S1 AR Simscape : Record  FileSettingsInternal="{\"entries\":[{\"content\":{\"excelSettings\":{\"content\":{},\"type\":\"Streamout.ExcelSettings\"}},\"type\":\"Streamout.FileSettingStorage\",\"uuid\":\"0ea696ca-752a-4f49-aa19-aaf05f026397\"}],\"packageUris\":[\"http://schema.mathworks.com/mf0/streamout_blocks/R2020a\"],\"version\":\"1.0\"}"  Layout=[1 1]  SignalsInternal="{\"entries\":[{\"content\":{\"signals\":[{\"content\":{\"blockPath\":[\"RBDmodel/L5-S1 AR readings/L5-S1 AR Simscape\"],\"dimensions\":[1],\"domain\":\"RBDmodel/L5-S1 AR readings/L5-S1 AR Simscape\",\"lineColor\":\"#fe330a\",\"port\":1,\"sid\":[\"\"],\"signalID\":1488,\"signalName\":\"L5-S1 AR Simscape Rotation\"},\"type\":\"RecordBlkView.Signal\",\"uuid\":\"ba465026-cfdc-4642-bcb4-f3fd199b7fea\"},{\"content\":{\"blockPath\":[\"RBDmodel/L5-S1 AR readings/L5-S1 AR Simscape\"],\"dimensions\":[1],\"domain\":\"RBDmodel/L5-S1 AR readings/L5-S1 AR Simscape\",\"lineColor\":\"#22b573\",\"port\":2,\"sid\":[\"\"],\"signalID\":1492,\"signalName\":\"L5-S1 AR Simscape Moment\"},\"type\":\"RecordBlkView.Signal\",\"uuid\":\"b1173115-f5bd-46eb-808a-071073e95144\"}]},\"type\":\"RecordBlkView.InputSignals\",\"uuid\":\"29903597-1dd1-480b-a347-da1b973a308e\"}],\"packageUris\":[\"http://schema.mathworks.com/mf0/streamout_blocks/R2020a\"],\"version\":\"1.0\"}"  VisualizationBindings="{\"xyplotplugin\":{\"info\":[{\"series\":[],\"subplotID\":1}]}}"  CompatibilityTag=XY
  wires:
  L5-S1 AR Simscape Rotation/1 -> L5-S1 AR Simscape/1, L5-S1 AR Rotation/1
  L5-S1 AR Simscape Moment/1 -> L5-S1 AR Simscape/2, L5-S1 AR Moment/1

== system RBDmodel/L5-S1 FE readings ==
  L5-S1 FE Simscape Rotation : Inport
  L5-S1 FE Simscape Moment : Inport  Port=2
  L5-S1 FE M-R : Record  FileSettingsInternal="{\"entries\":[{\"content\":{\"excelSettings\":{\"content\":{},\"type\":\"Streamout.ExcelSettings\"}},\"type\":\"Streamout.FileSettingStorage\",\"uuid\":\"03ebff2b-1b06-4da9-8d86-58934dddd7ed\"}],\"packageUris\":[\"http://schema.mathworks.com/mf0/streamout_blocks/R2020a\"],\"version\":\"1.0\"}"  Layout=[1 1]  SignalsInternal="{\"entries\":[{\"content\":{\"signals\":[{\"content\":{\"blockPath\":[\"RBDmodel/L5-S1 FE readings/L5-S1 FE M-R\"],\"dimensions\":[1],\"domain\":\"RBDmodel/L5-S1 FE readings/L5-S1 FE M-R\",\"lineColor\":\"#0072bd\",\"port\":1,\"sid\":[\"\"],\"signalID\":1496,\"signalName\":\"L5-S1 FE Simscape Rotation\"},\"type\":\"RecordBlkView.Signal\",\"uuid\":\"4de246c2-4ec3-445e-a7f4-51b6bec595d7\"},{\"content\":{\"blockPath\":[\"RBDmodel/L5-S1 FE readings/L5-S1 FE M-R\"],\"dimensions\":[1],\"domain\":\"RBDmodel/L5-S1 FE readings/L5-S1 FE M-R\",\"lineColor\":\"#d95319\",\"port\":2,\"sid\":[\"\"],\"signalID\":1500,\"signalName\":\"L5-S1 FE Simscape Moment\"},\"type\":\"RecordBlkView.Signal\",\"uuid\":\"295ba822-db53-4380-ae64-c387ea1aa2a6\"}]},\"type\":\"RecordBlkView.InputSignals\",\"uuid\":\"a4f81142-2ad9-408a-84a4-ad7d96e47c79\"}],\"packageUris\":[\"http://schema.mathworks.com/mf0/streamout_blocks/R2020a\"],\"version\":\"1.0\"}"  VisualizationBindings="{\"xyplotplugin\":{\"info\":[{\"series\":[],\"subplotID\":1}]}}"  CompatibilityTag=XY
  L5-S1 FE Moment : Scope
  L5-S1 FE Rot : Scope
  wires:
  L5-S1 FE Simscape Rotation/1 -> L5-S1 FE M-R/1, L5-S1 FE Rot/1
  L5-S1 FE Simscape Moment/1 -> L5-S1 FE M-R/2, L5-S1 FE Moment/1

== system RBDmodel/L5-S1 LB readings ==
  L5-S1 LB Simscape Rotation : Inport
  L5-S1 LB Simscape Moment : Inport  Port=2
  L5-S1 LB Moment : Scope
  L5-S1 LB Rotation : Scope
  L5-S1 LB Simscape : Record  FileSettingsInternal="{\"entries\":[{\"content\":{\"excelSettings\":{\"content\":{},\"type\":\"Streamout.ExcelSettings\"}},\"type\":\"Streamout.FileSettingStorage\",\"uuid\":\"1fe1a201-205f-45ed-a2ea-47484a7c7520\"}],\"packageUris\":[\"http://schema.mathworks.com/mf0/streamout_blocks/R2020a\"],\"version\":\"1.0\"}"  Layout=[1 1]  SignalsInternal="{\"entries\":[{\"content\":{\"signals\":[{\"content\":{\"blockPath\":[\"RBDmodel/L5-S1 LB readings/L5-S1 LB Simscape\"],\"dimensions\":[1],\"domain\":\"RBDmodel/L5-S1 LB readings/L5-S1 LB Simscape\",\"lineColor\":\"#edb120\",\"port\":1,\"sid\":[\"\"],\"signalID\":1504,\"signalName\":\"L5-S1 LB Simscape Rotation\"},\"type\":\"RecordBlkView.Signal\",\"uuid\":\"42707560-b32d-4806-8fd0-ea69026f8abf\"},{\"content\":{\"blockPath\":[\"RBDmodel/L5-S1 LB readings/L5-S1 LB Simscape\"],\"dimensions\":[1],\"domain\":\"RBDmodel/L5-S1 LB readings/L5-S1 LB Simscape\",\"lineColor\":\"#7e2f8e\",\"port\":2,\"sid\":[\"\"],\"signalID\":1508,\"signalName\":\"L5-S1 LB Simscape Moment\"},\"type\":\"RecordBlkView.Signal\",\"uuid\":\"8deed115-e70a-4796-a6f4-b1ca71a3285c\"}]},\"type\":\"RecordBlkView.InputSignals\",\"uuid\":\"cdf64b7d-8856-4a31-9fbb-9a1267f93f1b\"}],\"packageUris\":[\"http://schema.mathworks.com/mf0/streamout_blocks/R2020a\"],\"version\":\"1.0\"}"  VisualizationBindings="{\"xyplotplugin\":{\"info\":[{\"series\":[],\"subplotID\":1}]}}"  CompatibilityTag=XY
  wires:
  L5-S1 LB Simscape Moment/1 -> L5-S1 LB Simscape/2, L5-S1 LB Moment/1
  L5-S1 LB Simscape Rotation/1 -> L5-S1 LB Simscape/1, L5-S1 LB Rotation/1

== system RBDmodel/Left ITL Readings ==
  In1 : Inport
  In2 : Inport  Port=2
  In3 : Inport  Port=3
  In4 : Inport  Port=4
  In5 : Inport  Port=5
  Left L1-L2 ITL force : Scope
  Left L2-L3 ITL force : Scope
  Left L4-L5 ITL force : Scope
  Left L5-S1 ITL force : Scope
  Let L3-L4 ITL force : Scope
  wires:
  In4/1 -> Left L4-L5 ITL force/1
  In1/1 -> Left L1-L2 ITL force/1
  In5/1 -> Let L3-L4 ITL force/1
  In3/1 -> Left L5-S1 ITL force/1
  In2/1 -> Left L2-L3 ITL force/1

== system RBDmodel/Muscle force inputs ==
  Area in mm^2 : Constant  Value=26819
  Constant : Constant  Value=100000
  Display : Display
  Divide : Product  Inputs=**/
  IAP in Pascals : Constant  Value=IAP_Pa
  Left Abdominal Muscle Force : Constant  Value=-LeftAbdominalMuscleForce
  Left Back Muscle Force : Constant  Value=-LeftBackMuscleForce
  Left Transverse1 Muscle Force : Constant  Value=-LeftTransverse1MuscleForce
  Left Transverse2 Muscle Force : Constant  Value=-LeftTransverse2MuscleForce
  Right Abdominal Muscle Force : Constant  Value=-RightAbdominalMuscleForce
  Right Back Muscle Force : Constant  Value=-RightBackMuscleForce
  Right Transverse1 Muscle Force : Constant  Value=-RightTransverse1MuscleForce
  Right Transverse2 Muscle Force : Constant  Value=-RightTransverse2MuscleForce
  Scope{1..8} (8 alike) : Scope
  Sum of Square of Forces : MATLAB Function  TreatAsAtomicUnit=on
  RightAbdominalMuscleForce : Outport
  LeftAbdominalMuscleForce : Outport  Port=2
  RightBackMuscleForce : Outport  Port=3
  LeftBackMuscleForce : Outport  Port=4
  RightTransverse1MuscleForce : Outport  Port=5
  RightTransverse2MuscleForce : Outport  Port=6
  LeftTransverse1MuscleForce : Outport  Port=7
  LeftTransverse2MuscleForce : Outport  Port=8
  wires:
  Left Transverse2 Muscle Force/1 -> LeftTransverse2MuscleForce/1, Scope8/1, Sum of Square of Forces/8(F8)  "LeftTransverse2MuscleForce"
  Left Abdominal Muscle Force/1 -> LeftAbdominalMuscleForce/1, Scope2/1, Sum of Square of Forces/2(F2)  "LeftAbdominalMuscleForce"
  Sum of Square of Forces/1(SumofSquareofForces) -> Display/1  "SumofSquareofForces"
  Area in mm^2/1 -> Divide/2
  Left Back Muscle Force/1 -> Sum of Square of Forces/4(F4), LeftBackMuscleForce/1, Scope4/1  "LeftBackMuscleForce"
  Divide/1 -> Sum of Square of Forces/9(IAP)
  Left Transverse1 Muscle Force/1 -> LeftTransverse1MuscleForce/1, Scope7/1, Sum of Square of Forces/6(F6)  "LeftTransverse1MuscleForce"
  Right Abdominal Muscle Force/1 -> RightAbdominalMuscleForce/1, Scope1/1, Sum of Square of Forces/1(F1)  "RightAbdominalMuscleForce"
  Right Back Muscle Force/1 -> RightBackMuscleForce/1, Scope3/1, Sum of Square of Forces/3(F3)  "RightBackMuscleForce"
  Right Transverse2 Muscle Force/1 -> RightTransverse2MuscleForce/1, Scope6/1, Sum of Square of Forces/5(F5)  "RightTransverse2MuscleForce"
  Right Transverse1 Muscle Force/1 -> RightTransverse1MuscleForce/1, Scope5/1, Sum of Square of Forces/7(F7)  "RightTransverse1MuscleForce"
  IAP in Pascals/1 -> Divide/1
  Constant/1 -> Divide/3

== system RBDmodel/Plumbline readings ==
  x : Inport
  y : Inport  Port=2
  z : Inport  Port=3
  Check X Bounds : checkpacklib/Check Custom Bounds  InstantiateOnLoad=on  enabled=off  stopWhenAssertionFail=off  export=off  ViewDlgPos=[983.4 172.2 510.4 379.2]  OpenViewOnLoad=off  LaunchViewOnOpen=off  TimeUnits=seconds  EnableUpperBound=on  UpperBoundTimes=[0 3]  UpperBoundAmplitudes=[2 2];  EnableLowerBound=on  LowerBoundTimes=[0 3]  LowerBoundAmplitudes=[-2 -2]
      settings: LibrarySourceBlock=sdolib/Signal Constraints/Check Custom Bounds
  Check Y Bounds : checkpacklib/Check Custom Bounds  InstantiateOnLoad=on  enabled=off  stopWhenAssertionFail=off  export=off  ViewDlgPos=[509 222 510 390]  OpenViewOnLoad=off  LaunchViewOnOpen=off  TimeUnits=seconds  EnableUpperBound=on  UpperBoundTimes=[0 3]  UpperBoundAmplitudes=[2 2];  EnableLowerBound=on  LowerBoundTimes=[0 3]  LowerBoundAmplitudes=[-2 -2]
      settings: LibrarySourceBlock=sdolib/Signal Constraints/Check Custom Bounds
  Plumbline X distance (cm) : Display
  Plumbline Y distance (cm) : Display
  Plumbline Z distance (cm) : Display
  T1 plumbline coordinates : Scope  NumInputPorts=3
  wires:
  x/1 -> Plumbline X distance (cm)/1, Check X Bounds/1, T1 plumbline coordinates/1
  z/1 -> Plumbline Z distance (cm)/1, T1 plumbline coordinates/3
  y/1 -> Plumbline Y distance (cm)/1, Check Y Bounds/1, T1 plumbline coordinates/2
